simulink model "saab93_electric"  (R2018a)
settings: Solver=VariableStepDiscrete  StartTime=0.0  StopTime=1220  RelTol=1e-3  EnableMultiTasking=on
undefined symbols (not defined in the file): DiscIntNeverNeededParam
libraries: qss_tb_library x6
settings Model: Creator=grauers  LastModifiedBy=Luís Miranda
settings DataIOCC: LimitDataPoints=on  SaveFormat=Array  SignalLoggingSaveFormat=ModelDataLogs
settings OptimizationCC: InitFltsAndDblsToZero=on  LifeSpan=inf
settings DebuggingCC: SaveWithParameterizedLinksMsg=none  UnderspecifiedInitializationDetection=Classic  MergeDetectMultiDrivingBlocksExec=none  SignalResolutionControl=TryResolveAllWithWarning  SolverPrmCheckMsg=warning  MultiTaskDSMMsg=warning  MultiTaskCondExecSysMsg=none  FcnCallInpInsideContextMsg=warning  SFUnexpectedBacktrackingDiag=warning  SFNoUnconditionalDefaultTransitionDiag=warning  SFExecutionAtInitializationDiag=none
settings HardwareCC: ProdBitPerPointer=32  ProdBitPerSizeT=32  ProdBitPerPtrDiffT=32  ProdLargestAtomicFloat=None  ProdIntDivRoundTo=Undefined  ProdEndianess=Unspecified  ProdWordSize=32  ProdHWDeviceType=32-bit Generic
settings ModelReferenceCC: PropagateSignalLabelsOutOfModel=off
settings CodeAppCC: StateflowObjectComments=on
settings GRTTargetCC: TargetFcnLib=ansi_tfl_tmw.mat  TargetLangStandard=C89/C90 (ANSI)  CombineOutputUpdateFcns=off  GRTInterface=on
settings ConfigComp: CovMetricSettings=dw  CovHtmlReporting=on  CovSaveCumulativeToWorkspaceVar=on  CovSaveSingleToWorkspaceVar=on  CovExternalEMLEnable=off

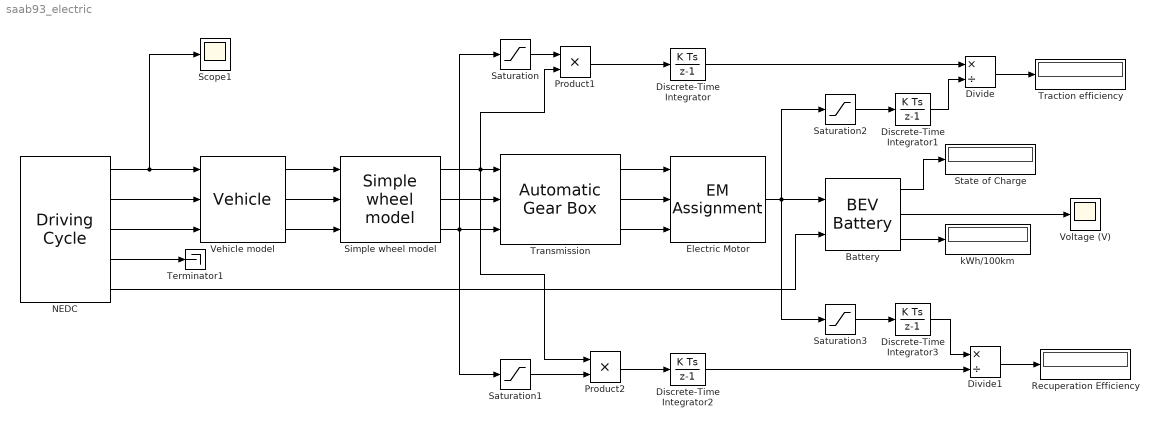
== system saab93_electric ==
  "Battery " : qss_tb_library/Energy Buffer/BEV Battery  Tag=battery  cell_series=100  cell_parallel=3  Q_BT_IC_rel=80
  Discrete-Time Integrator{,1..3} (4 alike) : DiscreteIntegrator  SampleTime=-1  ICPrevOutput=DiscIntNeverNeededParam  ICPrevScaledInput=DiscIntNeverNeededParam
  Divide : Product  Inputs=*/
  Divide1 : Product  Inputs=*/
  Electric Motor : qss_tb_library/Energy Converter/EM Assignment  P_em=115
  "NEDC " : qss_tb_library/Driving Cycle/Driving Cycle  Tag=cycle  cyclename1=NEDC  stepsize=1  autostop=on
  Product1 : Product
  Product2 : Product
  Recuperation Efficiency : Display
  Saturation : Saturate  UpperLimit=100000  LowerLimit=0
  Saturation1 : Saturate  UpperLimit=0  LowerLimit=-100000
  Saturation2 : Saturate  UpperLimit=100000  LowerLimit=0
  Saturation3 : Saturate  UpperLimit=0  LowerLimit=-100000
  Scope1 : Scope
  "Simple wheel model " : qss_tb_library/Vehicle/Simple wheel model  Tag=simple transmission  d_wheel=0.62
  State of Charge : Display
  Terminator1 : Terminator
  Traction efficiency : Display
  Transmission : qss_tb_library/Gear System/Automatic Gear Box  Tag=transmission  nog=1  i=[1]  i_diff=3.5  gearon=[]  gearoff=[]  d=0.62  e_GT=0.98  P_GT0=300  w_wheel_min=1
  "Vehicle model " : qss_tb_library/Vehicle/Vehicle  Tag=vehicle  m_f=1295+50+400  A_f=2  cw=0.30  mu=0.013  k_inertia=5
  Voltage (V) : Scope
  kWh/100km : Display
  wires:
  "NEDC "/4 -> Terminator1/1
  "NEDC "/1 -> Scope1/1, "Vehicle model "/1
  "NEDC "/2 -> "Vehicle model "/2
  "NEDC "/3 -> "Vehicle model "/3
  "Vehicle model "/1 -> "Simple wheel model "/1
  "Vehicle model "/2 -> "Simple wheel model "/2
  "Vehicle model "/3 -> "Simple wheel model "/3
  "Simple wheel model "/2 -> Transmission/2
  Transmission/1 -> Electric Motor/1
  Transmission/2 -> Electric Motor/2
  Transmission/3 -> Electric Motor/3
  Electric Motor/1 -> Saturation3/1, "Battery "/1, Saturation2/1
  "NEDC "/5 -> "Battery "/2
  "Battery "/2 -> Voltage (V)/1
  "Battery "/1 -> State of Charge/1
  "Battery "/3 -> kWh/100km/1
  Saturation/1 -> Product1/1
  Product1/1 -> Discrete-Time Integrator/1
  Saturation2/1 -> Discrete-Time Integrator1/1
  Discrete-Time Integrator1/1 -> Divide/2
  Discrete-Time Integrator/1 -> Divide/1
  Divide/1 -> Traction efficiency/1
  Divide1/1 -> Recuperation Efficiency/1
  Discrete-Time Integrator2/1 -> Divide1/2
  Discrete-Time Integrator3/1 -> Divide1/1
  Product2/1 -> Discrete-Time Integrator2/1
  Saturation1/1 -> Product2/2
  "Simple wheel model "/3 -> Saturation1/1, Transmission/3, Saturation/1
  "Simple wheel model "/1 -> Product2/1, Transmission/1, Product1/2
  Saturation3/1 -> Discrete-Time Integrator3/1
